simulink model "BT5_MophongtocdobangHT"  (R2022a)
settings: Solver=FixedStepAuto  StartTime=0.0  StopTime=20  FixedStep=0.01  RelTol=1e-3  EnableMultiTasking=on
settings Model: ExtModeTrigDuration=2  Creator=quoc2  LastModifiedBy=kietn
settings OptimizationCC: EnhancedBackFolding=on  PassReuseOutputArgsAs=Individual arguments  ZeroExternalMemoryAtStartup=off  ZeroInternalMemoryAtStartup=off  MaxStackSize=64  OptimizeBlockOrder=speed  DifferentSizesBufferReuse=on  EfficientTunableParamExpr=on
settings DebuggingCC: ParameterTunabilityLossMsg=error
settings HardwareCC: ProdBitPerPointer=32  ProdBitPerSizeT=32  ProdBitPerPtrDiffT=32  ProdLargestAtomicInteger=Long  ProdLargestAtomicFloat=Double  ProdWordSize=32  ProdHWDeviceType=ARM Compatible->ARM Cortex
settings SFSimCC: MATLABDynamicMemAlloc=off
settings RTWCC: SystemTargetFile=ert.tlc  HardwareBoard=ESP32-WROOM(Arduino Compatible)  TLCOptions="-aInlineSetEventsForThisBaseRateFcn=TLC_FALSE -aSuppressMultiTaskScheduler=TLC_FALSE              -aRateBasedStepFcn=0"  TemplateMakefile=ert_default_tmf  Toolchain=ESP32  BuildConfiguration=Faster Runs
settings CodeAppCC: ForceParamTrailComments=on  IgnoreCustomStorageClasses=off  OperatorAnnotations=on  SimulinkDataObjDesc=on  SFDataObjDesc=on  InsertBlockDesc=on
settings ERTTargetCC: SupportContinuousTime=on  SupportVariableSizeSignals=on  ExtMode=on  ExtModeTransport=3  ExtModeStaticAlloc=on  ExtModeStaticAllocSize=65536  ExtModeMexFile=ext_xcp  ExtModeMexArgs=0 3 921600 'E:\Matlab2022a\PID.elf' 3 1000  ExtModeIntrfLevel=Level2 - Open

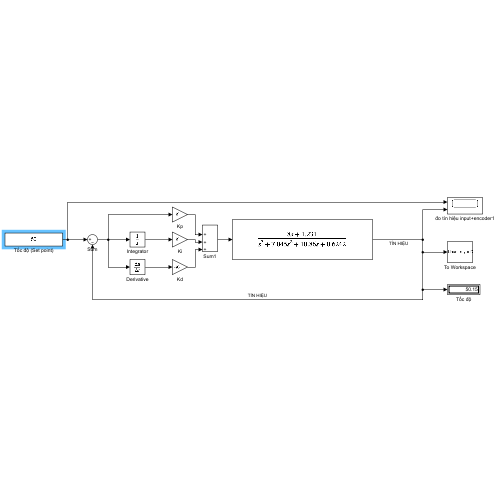
[thumbnail: Simulink's stored preview of the top-level diagram]
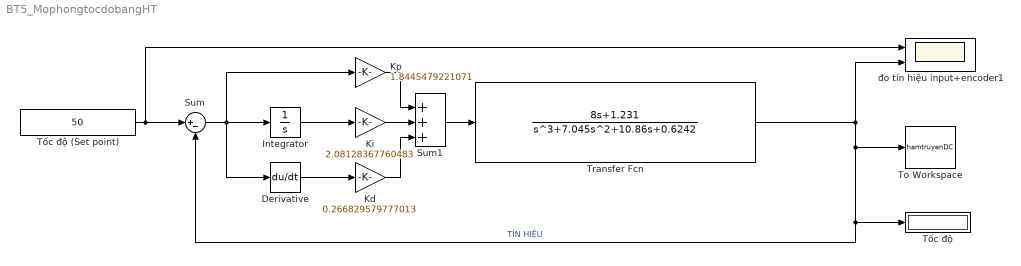
== system BT5_MophongtocdobangHT ==
  Derivative : Derivative
  Integrator : Integrator
  Kd : Gain  Gain=0.266829579777013
  Ki : Gain  Gain=2.08128367760483
  Kp : Gain  Gain=1.8445479221071
  Sum : Sum  Inputs=|+-
  Sum1 : Sum  Inputs=|+++
  To Workspace : ToWorkspace  VariableName=hamtruyenDC  SampleTime=-1
      settings: Save2DSignal=2-D array (concatenate along first dimension)
  Transfer Fcn : TransferFcn  Numerator=[8 1.231]  Denominator=[1 7.045 10.86 0.6242]
  Tốc độ : Display
  Tốc độ (Set point) : Constant  Value=50  VectorParams1D=off  OutMin=[-270]  OutMax=[270]  OutDataTypeStr=int16
  đo tín hiệu input+encoder1 : Scope  NumInputPorts=2
  wires:
  Transfer Fcn/1 -> đo tín hiệu input+encoder1/2, To Workspace/1, Sum/2, Tốc độ/1  "TÍN HIỆU"
  Tốc độ (Set point)/1 -> đo tín hiệu input+encoder1/1, Sum/1
  Sum/1 -> Derivative/1, Integrator/1, Kp/1
  Kp/1 -> Sum1/1
  Integrator/1 -> Ki/1
  Derivative/1 -> Kd/1
  Ki/1 -> Sum1/2
  Kd/1 -> Sum1/3
  Sum1/1 -> Transfer Fcn/1
